simulink model "swcStopLightsMgr"  (R2022b)
settings: Solver=FixedStepDiscrete  StartTime=0  StopTime=10.0  FixedStep=0.01  RelTol=1e-3
values from neighbouring files (symbols this model uses):
  C1d_stopLightsMgrPriorityTable = Simulink.Parameter    [swcStopLightsMgr_defineIntCalibs.m]
  C_stopLightsEmergencyPeriod = Simulink.Parameter    [swcStopLightsMgr_defineIntCalibs.m]
  C_stopLightsSpeedThresholdSafety = Simulink.Parameter    [swcBrakePedalSignalingApp_defineIntCalibs.m]    (also in swcStopLightsMgr_defineIntCalibs.m)
  CONST_TWO = uint8(2)    [swcStopLightsMgr_defineIntParams.m]
  failureAlert = Simulink.Signal    [swcStopLightsMgr_defineIntCalibs.m]
  Init_FailureAlert = struct('valueState',ValueState.VALUE_STATE_VALID,'failureAlert',FailureAlert.FAILURE_ALERT_NO,'occurrence',uint8(0))    [swcStopLightsMgr_defineIntParams.m]
  Init_lightRequest = struct('Left_lightState',StopLightStateID.STOP_LIGHT_STATE_ID_OFF,'Right_lightState',StopLightStateID.STOP_LIGHT_STATE_ID_OFF,'Middle_lightState',StopLightStateID.STOP_LIGHT_STATE_ID_OFF)    [swcStopLightsMgr_defineIntParams.m]
  Init_setLight = struct('usageId',uint8(0),'LightOut',Init_lightRequest,'requestedPattern',StopLightsPatternID.STOP_LIGHTS_PATTERN_ID_OFF,'isStopLightsOn',false,'BrakeLampStatus',CANBrakeLampStatus.CANBRAKELAMPSTATUS_OFF)    [swcStopLightsMgr_defineIntParams.m]
  Init_StopLightsEvent = struct('valueState',ValueState.VALUE_STATE_VALID,'usageId',uint8(0),'requestedPattern',StopLightsPatternID.STOP_LIGHTS_PATTERN_ID_OFF)    [swcStopLightsMgr_defineIntParams.m]
  Init_switchStopLightState = struct('lightState',StopLightStateID.STOP_LIGHT_STATE_ID_OFF)    [swcStopLightsMgr_defineIntParams.m]
  OCCURRENCE_FALSE = uint8(0)    [swcStopLightsMgr_defineIntParams.m]
  OCCURRENCE_TRUE = uint8(1)    [swcStopLightsMgr_defineIntParams.m]
  PeriodResolution = uint8(20)    [swcStopLightsMgr_defineIntParams.m]
  POWER_AUTHORIZER = uint8(1)    [swcStopLightsMgr_defineIntParams.m]
  STEP_StopLightsMgr = 0.01    [swcStopLightsMgr_defineIntParams.m]
  STOPLIGHTS_IDX = uint8(64)    [swcStopLightsMgr_defineIntParams.m]
  STOPLIGHTS_USAGES_OUTSIDE_WARNING_ON_STRONG_BRAKING = uint8(18)    [swcStopLightsMgr_defineIntParams.m]
  TENMs = uint8(10)    [swcStopLightsMgr_defineIntParams.m]
  USAGEID_DEF = uint8(255)    [swcStopLightsMgr_defineIntParams.m]
  USAGEID_MIN = uint8(0)    [swcStopLightsMgr_defineIntParams.m]
undefined symbols (not defined in the file or in its folder): CANBrakeLampStatus, CANStopLampDiagnosis, occurrence, StopLampDiagnosis, UsageAction, valueState, ValueState
libraries: Ampere_Library x27, simulink x3, KPIT_eBody_Lib_Lighting x1
(part 1 of 2)
settings Model: ModifiedByFormat=Smrithi Pai  Creator=Smrithi Pai  LastModifiedBy=Smrithi Pai
settings DataIOCC: SaveOutput=off  SignalLogging=off  DSMLogging=off  SaveTime=off  ReturnWorkspaceOutputs=off
settings OptimizationCC: DefaultParameterBehavior=Inlined  EnhancedBackFolding=on  PassReuseOutputArgsAs=Individual arguments  ZeroExternalMemoryAtStartup=off  ZeroInternalMemoryAtStartup=off  LifeSpan=inf  OptimizeBlockOrder=speed  DifferentSizesBufferReuse=on  OptimizationCustomize=off  EfficientTunableParamExpr=on
settings DebuggingCC: SignalInfNanChecking=error  SignalRangeChecking=error  ReadBeforeWriteMsg=EnableAllAsError  WriteAfterWriteMsg=EnableAllAsError  WriteAfterReadMsg=EnableAllAsError  AlgebraicLoopMsg=error  ArtificialAlgebraicLoopMsg=error  SaveWithDisabledLinksMsg=error  SaveWithParameterizedLinksMsg=error  BlockPriorityViolationMsg=error  MinStepSizeMsg=error  TimeAdjustmentMsg=warning  SolverPrmCheckMsg=error  MultiTaskRateTransMsg=warning  SingleTaskRateTransMsg=warning  TasksWithSamePriorityMsg=error  SigSpecEnsureSampleTimeMsg=error  CheckMatrixSingularityMsg=error  IntegerOverflowMsg=error  ParameterUnderflowMsg=error  ParameterPrecisionLossMsg=error  ParameterTunabilityLossMsg=error  FixptConstUnderflowMsg=warning  FixptConstOverflowMsg=warning  FixptConstPrecisionLossMsg=warning  UnderSpecifiedDataTypeMsg=error  UnnecessaryDatatypeConvMsg=warning  VectorMatrixConversionMsg=error  UnconnectedInputMsg=error  UnconnectedOutputMsg=error  UnconnectedLineMsg=error  FrameProcessingCompatibilityMsg=warning  UniqueDataStoreMsg=error  BusObjectLabelMismatch=error  RootOutportRequireBusObject=error  AssertControl=DisableAll  ModelReferenceIOMsg=error  UnknownTsInhSupMsg=error  ModelReferenceDataLoggingMessage=error  StateNameClashWarn=warning  StrictBusMsg=ErrorOnBusTreatedAsVector  NonBusSignalsTreatedAsBus=error  SFUnusedDataAndEventsDiag=error  SFInvalidInputDataAccessInChartInitDiag=error  SFTransitionOutsideNaturalParentDiag=error  SFUnreachableExecutionPathDiag=error  SFUndirectedBroadcastEventsDiag=error  SFTransitionActionBeforeConditionDiag=error  SFTemporalDelaySmallerThanSampleTimeDiag=error  SFSelfTransitionDiag=error  UnderSpecifiedDimensionMsg=error  VariantConditionMismatch=error
settings ModelReferenceCC: EnableRefExpFcnMdlSchedulingChecks=on  ModelReferenceNumInstancesAllowed=Single
settings SFSimCC: SimIntegrity=alwaysOn  SimGenImportedTypeDefs=on  CompileTimeRecursionLimit=0  EnableRuntimeRecursion=off  MATLABDynamicMemAlloc=off
settings RTWCC: Description=AUTOSAR  SystemTargetFile=autosar.tlc  GenCodeOnly=on  TemplateMakefile=ert_default_tmf
settings CodeAppCC: ForceParamTrailComments=on  IgnoreCustomStorageClasses=off  OperatorAnnotations=on  SimulinkDataObjDesc=on  SFDataObjDesc=on  InsertBlockDesc=on
settings STFCustomTargetCC: TargetLangStandard=C99 (ISO)  MultiwordLength=256  ParMdlRefBuildCompliant=on  CompOptLevelCompliant=on  IncludeMdlTerminateFcn=off  CombineOutputUpdateFcns=on  SuppressErrorStatus=on  ERTCustomFileBanners=on  SupportNonFinite=off  SupportComplex=off  SupportContinuousTime=off  SupportNonInlinedSFcns=off  RemoveResetFunc=on  MATLABClassNameForMDSCustomization=Simulink.SoftwareTarget.ERTCustomization  AutosarCompliant=on  UseToolchainInfoCompliant=on  LookupTableObjectStructAxisOrder=2,1,3,4,...  LUTObjectStructOrderEvenSpacing=Size,Table,Breakpoints  SystemTargetFile=autosar.tlc
settings ERTTargetCC: TargetLangStandard=C99 (ISO)  ConcurrentExecutionCompliant=off  IncludeMdlTerminateFcn=off  SuppressErrorStatus=on  SupportNonFinite=off  SupportComplex=off  ModelStepFunctionPrototypeControlCompliant=off  CPPClassGenCompliant=off  AutosarCompliant=on  LookupTableObjectStructAxisOrder=2,1,3,4,...  LUTObjectStructOrderEvenSpacing=Size,Table,Breakpoints  InlinedParameterPlacement=NonHierarchical  ERTCustomFileTemplate=example_file_process.tlc

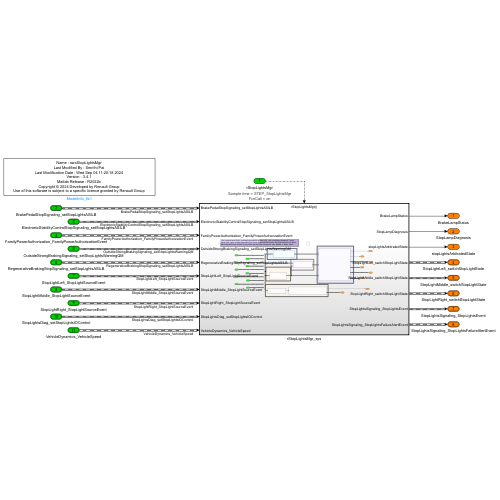
[thumbnail: Simulink's stored preview of the top-level diagram]
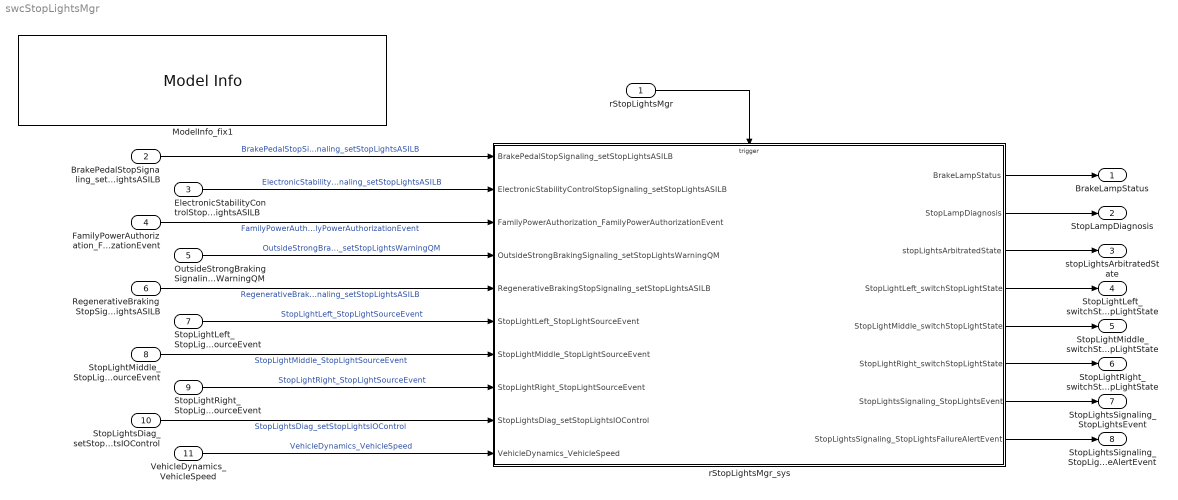
== system swcStopLightsMgr ==
  rStopLightsMgr : Inport  SampleTime=STEP_StopLightsMgr  OutputFunctionCall=on
      settings: AttributesFormatString=Sample time = %<SampleTime>\nFcnCall = %<OutputFunctionCall>
  BrakePedalStopSignaling_setStopLightsASILB : Inport  Port=2  OutDataTypeStr=Bus: setStopLightsASILB  PortDimensions=1  BusOutputAsStruct=on
  ElectronicStabilityControlStopSignaling_setStopLightsASILB : Inport  Port=3  OutDataTypeStr=Bus: setStopLightsASILB  PortDimensions=1  BusOutputAsStruct=on
  FamilyPowerAuthorization_FamilyPowerAuthorizationEvent : Inport  Port=4  OutDataTypeStr=Bus: FamilyPowerAuthorizationEvent  PortDimensions=1  BusOutputAsStruct=on
  OutsideStrongBrakingSignaling_setStopLightsWarningQM : Inport  Port=5  OutDataTypeStr=Bus: setStopLightsWarningQM  PortDimensions=1  BusOutputAsStruct=on
  RegenerativeBrakingStopSignaling_setStopLightsASILB : Inport  Port=6  OutDataTypeStr=Bus: setStopLightsASILB  PortDimensions=1  BusOutputAsStruct=on
  StopLightLeft_StopLightSourceEvent : Inport  Port=7  OutDataTypeStr=Bus: StopLightSourceEvent  PortDimensions=1  BusOutputAsStruct=on
  StopLightMiddle_StopLightSourceEvent : Inport  Port=8  OutDataTypeStr=Bus: StopLightSourceEvent  PortDimensions=1  BusOutputAsStruct=on
  StopLightRight_StopLightSourceEvent : Inport  Port=9  OutDataTypeStr=Bus: StopLightSourceEvent  PortDimensions=1  BusOutputAsStruct=on
  StopLightsDiag_setStopLightsIOControl : Inport  Port=10  OutDataTypeStr=Bus: setStopLightsIOControl  PortDimensions=1  BusOutputAsStruct=on
  VehicleDynamics_VehicleSpeed : Inport  Port=11  OutDataTypeStr=Bus: VehicleSpeed  PortDimensions=1  BusOutputAsStruct=on
  ModelInfo_fix1 : simulink/Model-Wide Utilities/Model Info  Frame=on  DisplayStringWithTags=|  HorizontalTextAlignment=Center  LeftAlignmentValue=0.5
      | Name : %<ModelName>
      | Last Modified By : %<LastModifiedBy>
      | Last Modification Date : %<LastModificationDate>
      | Version : %<ModelVersion>
      | Matlab Release : R2022b
      | Copyright © 2024 Developed by Renault Group
      | Use of this software is subject to a specific licence granted by Renault Group
  rStopLightsMgr_sys : Subsystem
  BrakeLampStatus : Outport  OutDataTypeStr=Enum: CANBrakeLampStatus  PortDimensions=1
  StopLampDiagnosis : Outport  Port=2  OutDataTypeStr=Enum: CANStopLampDiagnosis  PortDimensions=1
  stopLightsArbitratedState : Outport  Port=3  OutDataTypeStr=boolean  PortDimensions=1
  StopLightLeft_switchStopLightState : Outport  Port=4  OutDataTypeStr=Bus: switchStopLightState  PortDimensions=1  BusOutputAsStruct=on
  StopLightMiddle_switchStopLightState : Outport  Port=5  OutDataTypeStr=Bus: switchStopLightState  PortDimensions=1  BusOutputAsStruct=on
  StopLightRight_switchStopLightState : Outport  Port=6  OutDataTypeStr=Bus: switchStopLightState  PortDimensions=1  BusOutputAsStruct=on
  StopLightsSignaling_StopLightsEvent : Outport  Port=7  OutDataTypeStr=Bus: StopLightsEvent  PortDimensions=1  BusOutputAsStruct=on
  StopLightsSignaling_StopLightsFailureAlertEvent : Outport  Port=8  OutDataTypeStr=Bus: StopLightsFailureAlertEvent  PortDimensions=1  BusOutputAsStruct=on
  wires:
  rStopLightsMgr_sys/8(StopLightsSignaling_StopLightsFailureAlertEvent) -> StopLightsSignaling_StopLightsFailureAlertEvent/1
  rStopLightsMgr_sys/5(StopLightMiddle_switchStopLightState) -> StopLightMiddle_switchStopLightState/1
  rStopLightsMgr_sys/4(StopLightLeft_switchStopLightState) -> StopLightLeft_switchStopLightState/1
  rStopLightsMgr_sys/2(StopLampDiagnosis) -> StopLampDiagnosis/1
  rStopLightsMgr_sys/7(StopLightsSignaling_StopLightsEvent) -> StopLightsSignaling_StopLightsEvent/1
  rStopLightsMgr/1 -> rStopLightsMgr_sys/Trigger
  ElectronicStabilityControlStopSignaling_setStopLightsASILB/1 -> rStopLightsMgr_sys/2(ElectronicStabilityControlStopSignaling_setStopLightsASILB)  "ElectronicStabilityControlStopSignaling_setStopLightsASILB"
  FamilyPowerAuthorization_FamilyPowerAuthorizationEvent/1 -> rStopLightsMgr_sys/3(FamilyPowerAuthorization_FamilyPowerAuthorizationEvent)  "FamilyPowerAuthorization_FamilyPowerAuthorizationEvent"
  rStopLightsMgr_sys/3(stopLightsArbitratedState) -> stopLightsArbitratedState/1
  RegenerativeBrakingStopSignaling_setStopLightsASILB/1 -> rStopLightsMgr_sys/5(RegenerativeBrakingStopSignaling_setStopLightsASILB)  "RegenerativeBrakingStopSignaling_setStopLightsASILB"
  rStopLightsMgr_sys/1(BrakeLampStatus) -> BrakeLampStatus/1
  BrakePedalStopSignaling_setStopLightsASILB/1 -> rStopLightsMgr_sys/1(BrakePedalStopSignaling_setStopLightsASILB)  "BrakePedalStopSignaling_setStopLightsASILB"
  OutsideStrongBrakingSignaling_setStopLightsWarningQM/1 -> rStopLightsMgr_sys/4(OutsideStrongBrakingSignaling_setStopLightsWarningQM)  "OutsideStrongBrakingSignaling_setStopLightsWarningQM"
  StopLightLeft_StopLightSourceEvent/1 -> rStopLightsMgr_sys/6(StopLightLeft_StopLightSourceEvent)  "StopLightLeft_StopLightSourceEvent"
  StopLightMiddle_StopLightSourceEvent/1 -> rStopLightsMgr_sys/7(StopLightMiddle_StopLightSourceEvent)  "StopLightMiddle_StopLightSourceEvent"
  StopLightRight_StopLightSourceEvent/1 -> rStopLightsMgr_sys/8(StopLightRight_StopLightSourceEvent)  "StopLightRight_StopLightSourceEvent"
  StopLightsDiag_setStopLightsIOControl/1 -> rStopLightsMgr_sys/9(StopLightsDiag_setStopLightsIOControl)  "StopLightsDiag_setStopLightsIOControl"
  rStopLightsMgr_sys/6(StopLightRight_switchStopLightState) -> StopLightRight_switchStopLightState/1
  VehicleDynamics_VehicleSpeed/1 -> rStopLightsMgr_sys/10(VehicleDynamics_VehicleSpeed)  "VehicleDynamics_VehicleSpeed"

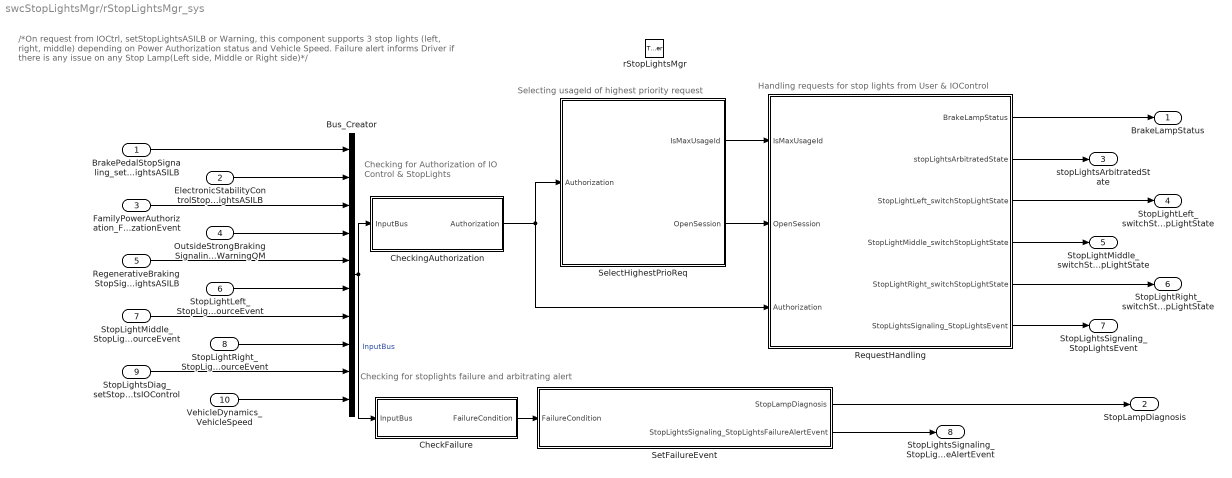
== system swcStopLightsMgr/rStopLightsMgr_sys ==
  note: Checking for Authorization of
      | IO Control & StopLights
  note: Handling requests for stop lights from User & IOControl
  note: Checking for stoplights failure and arbitrating alert
  note: Selecting usageId of highest priority request
  note: /*On request from IOCtrl, setStopLightsASILB or Warning, this component supports 3 stop lights (left, right, middle) depending on Power Authorization status and Vehicle Speed. Failure alert informs Driver if there is any issue on any Stop Lamp(Left side, Middle or Right side)*/
  BrakePedalStopSignaling_setStopLightsASILB : Inport
  ElectronicStabilityControlStopSignaling_setStopLightsASILB : Inport  Port=2
  FamilyPowerAuthorization_FamilyPowerAuthorizationEvent : Inport  Port=3
  OutsideStrongBrakingSignaling_setStopLightsWarningQM : Inport  Port=4
  RegenerativeBrakingStopSignaling_setStopLightsASILB : Inport  Port=5
  StopLightLeft_StopLightSourceEvent : Inport  Port=6
  StopLightMiddle_StopLightSourceEvent : Inport  Port=7
  StopLightRight_StopLightSourceEvent : Inport  Port=8
  StopLightsDiag_setStopLightsIOControl : Inport  Port=9
  VehicleDynamics_VehicleSpeed : Inport  Port=10
  rStopLightsMgr : TriggerPort  TriggerType=function-call  VariantControl=(inherit)  SampleTimeType=periodic  SampleTime=-1  PortDimensions=1
      settings: AttributesFormatString=%<StatesWhenEnabling>\n
  Bus_Creator : BusCreator  Inputs=10
  CheckFailure : Subsystem  Description=|  TreatAsAtomicUnit=on
      | StopLightsMgr_Req_41
      | StopLightsMgr_Req_43
      | StopLightsMgr_Req_100333
  CheckingAuthorization : Subsystem  Description=StopLightsMgr_Req_22  TreatAsAtomicUnit=on
  RequestHandling : Subsystem  Description=<binary blob, 146 chars, not shown>  TreatAsAtomicUnit=on
  SelectHighestPrioReq : Subsystem  Description=StopLightsMgr_Req_22  TreatAsAtomicUnit=on
  SetFailureEvent : Subsystem  Description=|  TreatAsAtomicUnit=on
      | StopLightsMgr_Req_40
      | StopLightsMgr_Req_44
      | StopLightsMgr_Req_48
      | StopLightsMgr_Req_49
  BrakeLampStatus : Outport  InitialOutput=CANBrakeLampStatus.CANBRAKELAMPSTATUS_OFF
      settings: AttributesFormatString=Init = %<InitialOutput>\n
  StopLampDiagnosis : Outport  Port=2  InitialOutput=CANStopLampDiagnosis.CANSTOPLAMPDIAGNOSIS_NO_FAILURE
      settings: AttributesFormatString=Init = %<InitialOutput>\n
  stopLightsArbitratedState : Outport  Port=3  InitialOutput=false
      settings: AttributesFormatString=Init = %<InitialOutput>\n
  StopLightLeft_switchStopLightState : Outport  Port=4  InitialOutput=Init_switchStopLightState
      settings: AttributesFormatString=Init = %<InitialOutput>\n
  StopLightMiddle_switchStopLightState : Outport  Port=5  InitialOutput=Init_switchStopLightState
      settings: AttributesFormatString=Init = %<InitialOutput>\n
  StopLightRight_switchStopLightState : Outport  Port=6  InitialOutput=Init_switchStopLightState
      settings: AttributesFormatString=Init = %<InitialOutput>\n
  StopLightsSignaling_StopLightsEvent : Outport  Port=7  InitialOutput=Init_StopLightsEvent
      settings: AttributesFormatString=Init = %<InitialOutput>\n
  StopLightsSignaling_StopLightsFailureAlertEvent : Outport  Port=8  InitialOutput=Init_FailureAlert
      settings: AttributesFormatString=Init = %<InitialOutput>\n
  wires:
  BrakePedalStopSignaling_setStopLightsASILB/1 -> Bus_Creator/1
  ElectronicStabilityControlStopSignaling_setStopLightsASILB/1 -> Bus_Creator/2
  FamilyPowerAuthorization_FamilyPowerAuthorizationEvent/1 -> Bus_Creator/3
  OutsideStrongBrakingSignaling_setStopLightsWarningQM/1 -> Bus_Creator/4
  RegenerativeBrakingStopSignaling_setStopLightsASILB/1 -> Bus_Creator/5
  StopLightLeft_StopLightSourceEvent/1 -> Bus_Creator/6
  StopLightMiddle_StopLightSourceEvent/1 -> Bus_Creator/7
  StopLightRight_StopLightSourceEvent/1 -> Bus_Creator/8
  StopLightsDiag_setStopLightsIOControl/1 -> Bus_Creator/9
  VehicleDynamics_VehicleSpeed/1 -> Bus_Creator/10
  RequestHandling/1(BrakeLampStatus) -> BrakeLampStatus/1
  SelectHighestPrioReq/1(IsMaxUsageId) -> RequestHandling/1(IsMaxUsageId)
  CheckingAuthorization/1(Authorization) -> RequestHandling/3(Authorization), SelectHighestPrioReq/1(Authorization)
  RequestHandling/2(stopLightsArbitratedState) -> stopLightsArbitratedState/1
  RequestHandling/3(StopLightLeft_switchStopLightState) -> StopLightLeft_switchStopLightState/1
  RequestHandling/4(StopLightMiddle_switchStopLightState) -> StopLightMiddle_switchStopLightState/1
  RequestHandling/5(StopLightRight_switchStopLightState) -> StopLightRight_switchStopLightState/1
  RequestHandling/6(StopLightsSignaling_StopLightsEvent) -> StopLightsSignaling_StopLightsEvent/1
  SetFailureEvent/1(StopLampDiagnosis) -> StopLampDiagnosis/1
  SetFailureEvent/2(StopLightsSignaling_StopLightsFailureAlertEvent) -> StopLightsSignaling_StopLightsFailureAlertEvent/1
  Bus_Creator/1 -> CheckFailure/1(InputBus), CheckingAuthorization/1(InputBus)  "InputBus"
  CheckFailure/1(FailureCondition) -> SetFailureEvent/1(FailureCondition)
  SelectHighestPrioReq/2(OpenSession) -> RequestHandling/2(OpenSession)

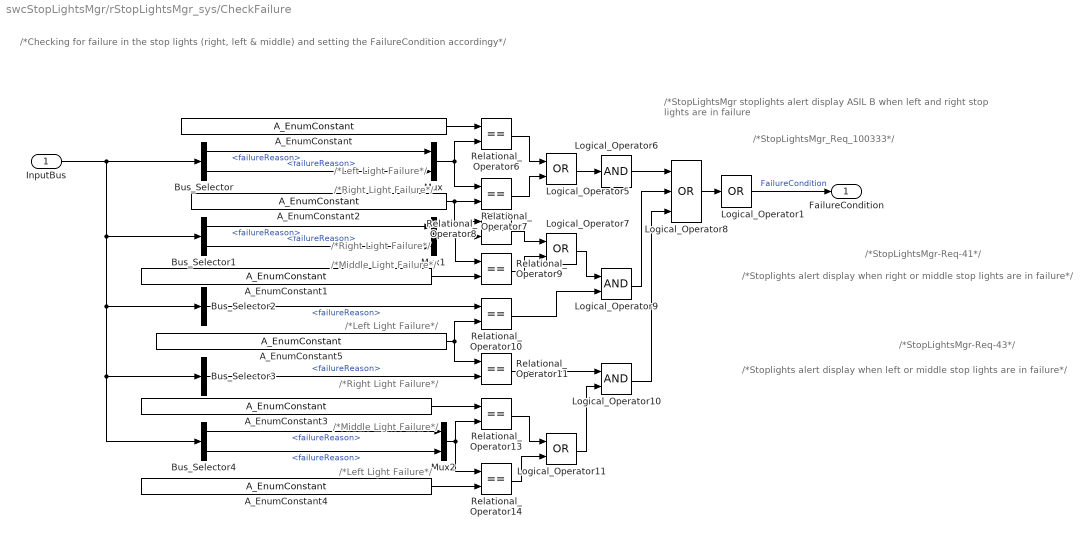
== system swcStopLightsMgr/rStopLightsMgr_sys/CheckFailure ==
  note: /*Left Light Failure*/
  note: /*Stoplights alert display when right or middle stop
      | lights are in failure*/
  note: /*StopLightsMgr stoplights alert display
      | ASIL B when left and right stop lights are in failure
  note: /*Stoplights alert display when left or middle stop lights
      | are in failure*/
  note: /*Right Light Failure*/
  note: /*Right Light Failure*/
  note: /*Middle Light Failure*/
  note: /*Left Light Failure*/
  note: /*Middle Light Failure*/
  note: /*Left Light Failure*/
  note: /*Right Light Failure*/
  note: /*StopLightsMgr_Req_100333*/
  note: /*StopLightsMgr-Req-41*/
  note: /*StopLightsMgr-Req-43*/
  note: /*Checking for failure in the stop lights (right, left & middle) and setting the FailureCondition accordingy*/
  InputBus : Inport
  A_EnumConstant : Ampere_Library/User_Defined_Libraries/Sources/A_EnumConstant  Tag=[LIB]  OutDataTypeStr=Enum: LightSourceFailureReason  EnumVal=LIGHT_SOURCE_FAILURE_REASON_SC_TO_GND
      settings: AttributesFormatString=Enum: LightSourceFailureReason
  A_EnumConstant1 : Ampere_Library/User_Defined_Libraries/Sources/A_EnumConstant  Tag=[LIB]  OutDataTypeStr=Enum: LightSourceFailureReason  EnumVal=LIGHT_SOURCE_FAILURE_REASON_SC_TO_GND
      settings: AttributesFormatString=Enum: LightSourceFailureReason
  A_EnumConstant2 : Ampere_Library/User_Defined_Libraries/Sources/A_EnumConstant  Tag=[LIB]  OutDataTypeStr=Enum: LightSourceFailureReason  EnumVal=LIGHT_SOURCE_FAILURE_REASON_OPEN_CIRCUIT
      settings: AttributesFormatString=Enum: LightSourceFailureReason
  A_EnumConstant3 : Ampere_Library/User_Defined_Libraries/Sources/A_EnumConstant  Tag=[LIB]  OutDataTypeStr=Enum: LightSourceFailureReason  EnumVal=LIGHT_SOURCE_FAILURE_REASON_OPEN_CIRCUIT
      settings: AttributesFormatString=Enum: LightSourceFailureReason
  A_EnumConstant4 : Ampere_Library/User_Defined_Libraries/Sources/A_EnumConstant  Tag=[LIB]  OutDataTypeStr=Enum: LightSourceFailureReason  EnumVal=LIGHT_SOURCE_FAILURE_REASON_SC_TO_GND
      settings: AttributesFormatString=Enum: LightSourceFailureReason
  A_EnumConstant5 : Ampere_Library/User_Defined_Libraries/Sources/A_EnumConstant  Tag=[LIB]  OutDataTypeStr=Enum: LightSourceFailureReason  EnumVal=LIGHT_SOURCE_FAILURE_REASON_NONE
      settings: AttributesFormatString=Enum: LightSourceFailureReason
  Bus_Selector : BusSelector  OutputSignals=StopLightLeft_StopLightSourceEvent.failureReason,StopLightRight_StopLightSourceEvent.failureReason
  Bus_Selector1 : BusSelector  OutputSignals=StopLightMiddle_StopLightSourceEvent.failureReason,StopLightRight_StopLightSourceEvent.failureReason
  Bus_Selector2 : BusSelector  OutputSignals=StopLightLeft_StopLightSourceEvent.failureReason
  Bus_Selector3 : BusSelector  OutputSignals=StopLightRight_StopLightSourceEvent.failureReason
  Bus_Selector4 : BusSelector  OutputSignals=StopLightMiddle_StopLightSourceEvent.failureReason,StopLightLeft_StopLightSourceEvent.failureReason
  Logical_Operator1 : Logic  Operator=OR  Inputs=1  OutDataTypeStr=boolean
  Logical_Operator10 : Logic  OutDataTypeStr=boolean
  Logical_Operator11 : Logic  Operator=OR  OutDataTypeStr=boolean
  Logical_Operator5 : Logic  Operator=OR  OutDataTypeStr=boolean
  Logical_Operator6 : Logic  Inputs=1  OutDataTypeStr=boolean
  Logical_Operator7 : Logic  Operator=OR  OutDataTypeStr=boolean
  Logical_Operator8 : Logic  Operator=OR  Inputs=3  OutDataTypeStr=boolean
  Logical_Operator9 : Logic  OutDataTypeStr=boolean
  Mux : Mux  Inputs=2
  Mux1 : Mux  Inputs=2
  Mux2 : Mux  Inputs=2
  Relational_Operator{6..11,13..14} (8 alike) : RelationalOperator  Operator===  OutDataTypeStr=boolean  RndMeth=Zero
  FailureCondition : Outport
  wires:
  Relational_Operator11/1 -> Logical_Operator10/1
  Mux/1 -> Relational_Operator6/2, Relational_Operator7/1
  Bus_Selector4/1 -> Mux2/1  "<failureReason>"
  Bus_Selector1/2 -> Mux1/2  "<failureReason>"
  Logical_Operator6/1 -> Logical_Operator8/1
  InputBus/1 -> Bus_Selector/1, Bus_Selector4/1, Bus_Selector3/1, Bus_Selector2/1, Bus_Selector1/1
  Logical_Operator9/1 -> Logical_Operator8/2
  Relational_Operator7/1 -> Logical_Operator5/2
  Mux2/1 -> Relational_Operator14/1, Relational_Operator13/2
  Bus_Selector/2 -> Mux/2  "<failureReason>"
  A_EnumConstant2/1 -> Relational_Operator8/1, Relational_Operator7/2
  A_EnumConstant/1 -> Relational_Operator6/1
  Bus_Selector3/1 -> Relational_Operator11/2  "<failureReason>"
  Relational_Operator8/1 -> Logical_Operator7/1
  Mux1/1 -> Relational_Operator9/1, Relational_Operator8/2
  Logical_Operator5/1 -> Logical_Operator6/1
  A_EnumConstant1/1 -> Relational_Operator9/2
  A_EnumConstant5/1 -> Relational_Operator11/1, Relational_Operator10/2
  Bus_Selector2/1 -> Relational_Operator10/1  "<failureReason>"
  A_EnumConstant3/1 -> Relational_Operator13/1
  Bus_Selector/1 -> Mux/1  "<failureReason>"
  Relational_Operator10/1 -> Logical_Operator9/2
  Relational_Operator6/1 -> Logical_Operator5/1
  Bus_Selector1/1 -> Mux1/1  "<failureReason>"
  Relational_Operator9/1 -> Logical_Operator7/2
  Logical_Operator11/1 -> Logical_Operator10/2
  A_EnumConstant4/1 -> Relational_Operator14/2
  Bus_Selector4/2 -> Mux2/2  "<failureReason>"
  Logical_Operator10/1 -> Logical_Operator8/3
  Logical_Operator7/1 -> Logical_Operator9/1
  Relational_Operator14/1 -> Logical_Operator11/2
  Relational_Operator13/1 -> Logical_Operator11/1
  Logical_Operator8/1 -> Logical_Operator1/1
  Logical_Operator1/1 -> FailureCondition/1  "FailureCondition"

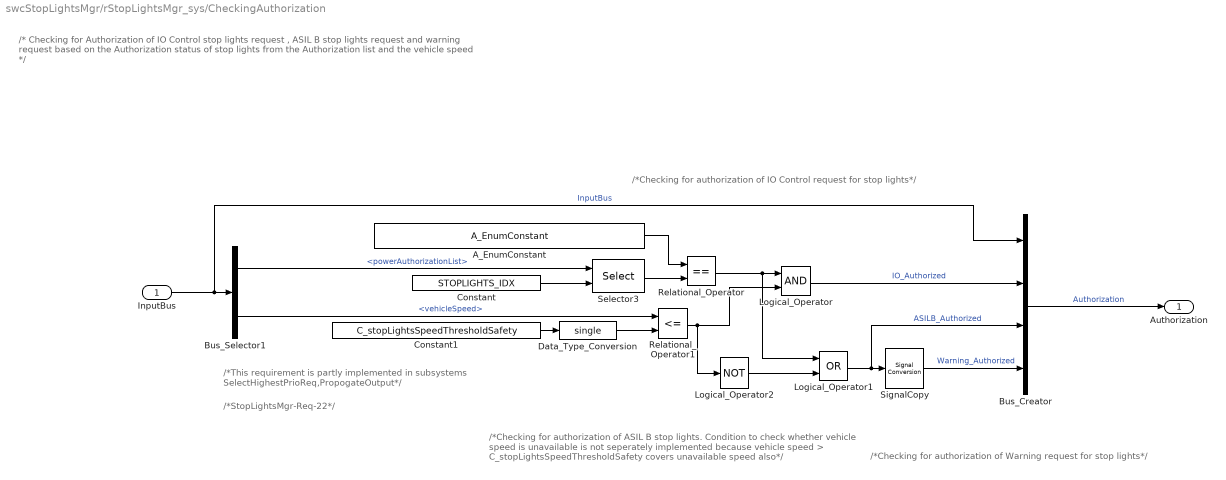
== system swcStopLightsMgr/rStopLightsMgr_sys/CheckingAuthorization ==
  note: /*Checking for authorization of ASIL B stop lights. Condition to check whether vehicle speed is unavailable is not seperately implemented because vehicle speed > C_stopLightsSpeedThresholdSafety covers unavailable speed also*/
  note: /*StopLightsMgr-Req-22*/
  note: /*This requirement is partly implemented in subsystems SelectHighestPrioReq,PropogateOutput*/
  note: /*Checking for authorization of IO Control request for stop lights*/
  note: /*Checking for authorization of Warning request for stop lights*/
  note: /* Checking for Authorization of IO Control stop lights request , ASIL B stop lights request and warning request based on the Authorization status of stop lights from the Authorization list and the vehicle speed */
  InputBus : Inport
  A_EnumConstant : Ampere_Library/User_Defined_Libraries/Sources/A_EnumConstant  Tag=[LIB]  OutDataTypeStr=Enum: PowerAuthorizationStatus  EnumVal=POWERAUTHORIZATIONSTATUS_AUTHORIZED
      settings: AttributesFormatString=Enum: PowerAuthorizationStatus
  Bus_Creator : BusCreator  Inputs=4
  Bus_Selector1 : BusSelector  OutputSignals=FamilyPowerAuthorization_FamilyPowerAuthorizationEvent.powerAuthorizationList,VehicleDynamics_VehicleSpeed.vehicleSpeed
  Constant : Constant  Value=STOPLIGHTS_IDX
  Constant1 : Constant  Value=C_stopLightsSpeedThresholdSafety
  Data_Type_Conversion : DataTypeConversion  OutDataTypeStr=single  SaturateOnIntegerOverflow=off
  Logical_Operator : Logic  OutDataTypeStr=boolean
  Logical_Operator1 : Logic  Operator=OR  OutDataTypeStr=boolean
  Logical_Operator2 : Logic  Operator=NOT  OutDataTypeStr=boolean
  Relational_Operator : RelationalOperator  Operator===  OutDataTypeStr=boolean  RndMeth=Zero
  Relational_Operator1 : RelationalOperator  Operator=<=  OutDataTypeStr=boolean  RndMeth=Zero
  Selector3 : Selector  IndexMode=Zero-based  InputPortWidth=450  IndexOptions=Index vector (port)  Indices=[1 3]  OutputSizes=1
      settings: AttributesFormatString=%<IndexMode>\n
  SignalCopy : SignalConversion  OverrideOpt=off
  Authorization : Outport
  wires:
  Bus_Selector1/1 -> Selector3/1  "<powerAuthorizationList>"
  A_EnumConstant/1 -> Relational_Operator/1
  Constant/1 -> Selector3/2
  Selector3/1 -> Relational_Operator/2
  InputBus/1 -> Bus_Creator/1, Bus_Selector1/1  "InputBus"
  Constant1/1 -> Data_Type_Conversion/1
  Data_Type_Conversion/1 -> Relational_Operator1/2
  Relational_Operator1/1 -> Logical_Operator2/1, Logical_Operator/2
  Bus_Selector1/2 -> Relational_Operator1/1  "<vehicleSpeed>"
  Relational_Operator/1 -> Logical_Operator/1, Logical_Operator1/1
  Logical_Operator2/1 -> Logical_Operator1/2
  Logical_Operator/1 -> Bus_Creator/2  "IO_Authorized"
  Logical_Operator1/1 -> Bus_Creator/3, SignalCopy/1  "ASILB_Authorized"
  SignalCopy/1 -> Bus_Creator/4  "Warning_Authorized"
  Bus_Creator/1 -> Authorization/1  "Authorization"

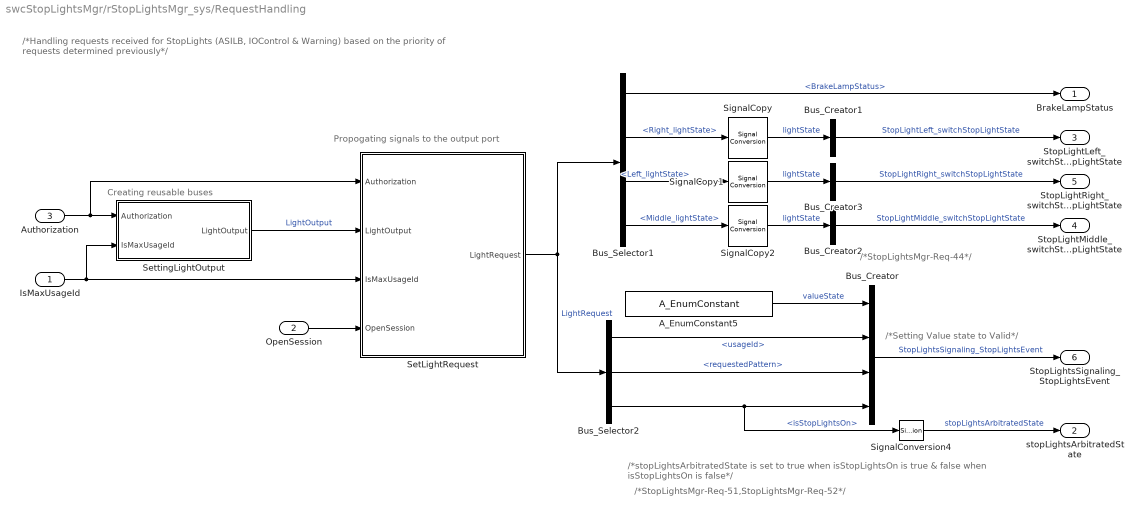
== system swcStopLightsMgr/rStopLightsMgr_sys/RequestHandling ==
  note: Propogating signals to the output port
  note: /*Setting Value state to Valid*/
  note: /*stopLightsArbitratedState is set to true when isStopLightsOn is true & false when isStopLightsOn is false*/
  note: /*StopLightsMgr-Req-44*/
  note: /*Handling requests received for StopLights (ASILB, IOControl & Warning) based on the priority of requests determined previously*/
  note: /*StopLightsMgr-Req-51,StopLightsMgr-Req-52*/
  note: Creating reusable buses
  IsMaxUsageId : Inport
  OpenSession : Inport  Port=2
  Authorization : Inport  Port=3
  A_EnumConstant5 : Ampere_Library/User_Defined_Libraries/Sources/A_EnumConstant  Tag=[LIB]  OutDataTypeStr=Enum: ValueState  EnumVal=VALUE_STATE_VALID
      settings: AttributesFormatString=Enum: ValueState
  Bus_Creator : BusCreator  Inputs='valueState','usageId','requestedPattern','isStopLightsOn'  OutDataTypeStr=Bus: StopLightsEvent  NonVirtualBus=on
  Bus_Creator1 : BusCreator  Inputs=lightState  OutDataTypeStr=Bus: switchStopLightState  NonVirtualBus=on
  Bus_Creator2 : BusCreator  Inputs=lightState  OutDataTypeStr=Bus: switchStopLightState  NonVirtualBus=on
  Bus_Creator3 : BusCreator  Inputs=lightState  OutDataTypeStr=Bus: switchStopLightState  NonVirtualBus=on
  Bus_Selector1 : BusSelector  OutputSignals=BrakeLampStatus,LightOut.Right_lightState,LightOut.Left_lightState,LightOut.Middle_lightState
  Bus_Selector2 : BusSelector  OutputSignals=usageId,requestedPattern,isStopLightsOn
  SetLightRequest : Subsystem  TreatAsAtomicUnit=on
  SettingLightOutput : Subsystem  Description=<binary blob, 196 chars, not shown>  TreatAsAtomicUnit=on
  SignalConversion4 : SignalConversion  OverrideOpt=off
  SignalCopy : SignalConversion  OverrideOpt=off
  SignalCopy1 : SignalConversion  OverrideOpt=off
  SignalCopy2 : SignalConversion  OverrideOpt=off
  BrakeLampStatus : Outport
  stopLightsArbitratedState : Outport  Port=2
  StopLightLeft_switchStopLightState : Outport  Port=3
  StopLightMiddle_switchStopLightState : Outport  Port=4
  StopLightRight_switchStopLightState : Outport  Port=5
  StopLightsSignaling_StopLightsEvent : Outport  Port=6
  wires:
  SetLightRequest/1(LightRequest) -> Bus_Selector1/1, Bus_Selector2/1  "LightRequest"
  Bus_Creator1/1 -> StopLightLeft_switchStopLightState/1  "StopLightLeft_switchStopLightState"
  Bus_Creator2/1 -> StopLightMiddle_switchStopLightState/1  "StopLightMiddle_switchStopLightState"
  Bus_Creator3/1 -> StopLightRight_switchStopLightState/1  "StopLightRight_switchStopLightState"
  SignalCopy1/1 -> Bus_Creator3/1  "lightState"
  Bus_Selector2/1 -> Bus_Creator/2  "<usageId>"
  Bus_Selector2/3 -> SignalConversion4/1, Bus_Creator/4  "<isStopLightsOn>"
  A_EnumConstant5/1 -> Bus_Creator/1  "valueState"
  Bus_Creator/1 -> StopLightsSignaling_StopLightsEvent/1  "StopLightsSignaling_StopLightsEvent"
  Bus_Selector2/2 -> Bus_Creator/3  "<requestedPattern>"
  SignalCopy2/1 -> Bus_Creator2/1  "lightState"
  SignalCopy/1 -> Bus_Creator1/1  "lightState"
  SettingLightOutput/1(LightOutput) -> SetLightRequest/2(LightOutput)  "LightOutput"
  SignalConversion4/1 -> stopLightsArbitratedState/1  "stopLightsArbitratedState"
  Bus_Selector1/2 -> SignalCopy/1  "<Right_lightState>"
  Bus_Selector1/3 -> SignalCopy1/1  "<Left_lightState>"
  Bus_Selector1/4 -> SignalCopy2/1  "<Middle_lightState>"
  Bus_Selector1/1 -> BrakeLampStatus/1  "<BrakeLampStatus>"
  IsMaxUsageId/1 -> SettingLightOutput/2(IsMaxUsageId), SetLightRequest/3(IsMaxUsageId)
  OpenSession/1 -> SetLightRequest/4(OpenSession)
  Authorization/1 -> SetLightRequest/1(Authorization), SettingLightOutput/1(Authorization)

== system swcStopLightsMgr/rStopLightsMgr_sys/SelectHighestPrioReq ==
  note: Selecting the UsageID of the client which has the highest
      | priority
  note: /*This requirement is partly implemented in subsystems
      | CheckingAuthorization, PropogateOutput*/
  note: Selecting the Usage ID depending on the request received StopLights, IO Control or
      | Warning
  note: /*StopLightsMgr-Req-22*/
  note: /* In this subsystem ASILB, IOCtrl and warning priority selection(Selected_Priority) is done. If there is no request fromASILB, IOCTRL and warning then stop lamps will turn off*/
  Authorization : Inport
  Bus_Selector2 : BusSelector  OutputSignals=IO_Authorized,ASILB_Authorized,Warning_Authorized
  SelectRequestFromPriority : Subsystem
  SelectingRequest : Subsystem  TreatAsAtomicUnit=on
  IsMaxUsageId : Outport
  OpenSession : Outport  Port=2
  wires:
  SelectingRequest/1(Selected_usageId) -> SelectRequestFromPriority/1(Selected_usageId)  "Selected_usageId"
  SelectRequestFromPriority/1(IsMaxUsageId) -> IsMaxUsageId/1  "IsMaxUsageId"
  SelectingRequest/2(InputUsageID) -> SelectRequestFromPriority/2(InputUsageID)
  Authorization/1 -> Bus_Selector2/1, SelectingRequest/1(Authorization)
  Bus_Selector2/2 -> SelectingRequest/3(ASILB_Authorized)  "<ASILB_Authorized>"
  Bus_Selector2/3 -> SelectingRequest/4(Warning_Authorized)  "<Warning_Authorized>"
  SelectingRequest/3(OpenSession) -> OpenSession/1  "OpenSession"
  Bus_Selector2/1 -> SelectingRequest/2(IO_Authorized)  "<IO_Authorized>"

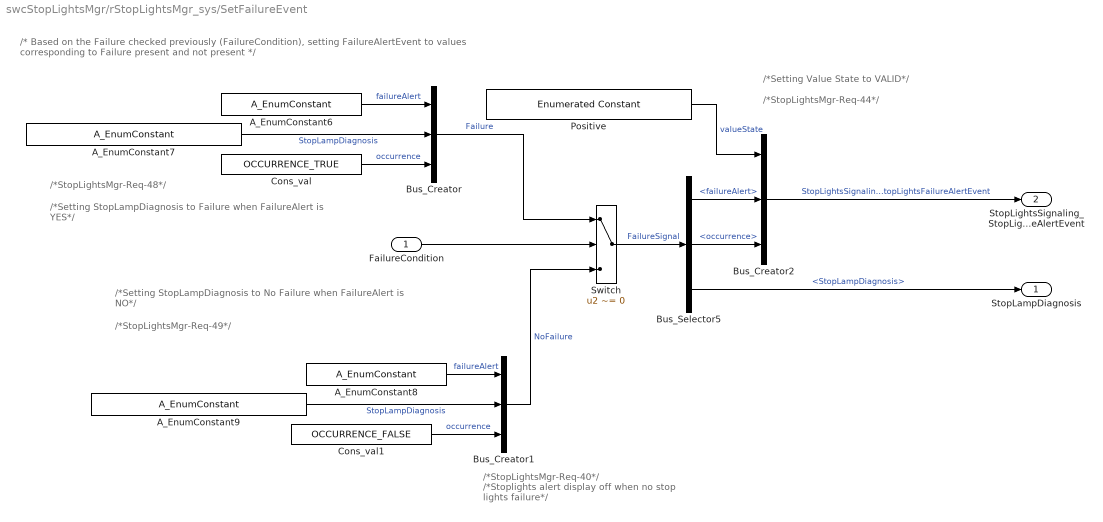
== system swcStopLightsMgr/rStopLightsMgr_sys/SetFailureEvent ==
  note: /*Setting Value State to VALID*/
  note: /*Setting StopLampDiagnosis to Failure
      | when FailureAlert is YES*/
  note: /*Stoplights alert display
      | off when no stop lights failure*/
  note: /*StopLightsMgr-Req-40*/
  note: /*StopLightsMgr-Req-44*/
  note: /*StopLightsMgr-Req-48*/
  note: /*StopLightsMgr-Req-49*/
  note: /*Setting StopLampDiagnosis to No Failure
      | when FailureAlert is NO*/
  note: /* Based on the Failure checked previously (FailureCondition), setting FailureAlertEvent to values corresponding to Failure present and not present */
  FailureCondition : Inport
  A_EnumConstant6 : Ampere_Library/User_Defined_Libraries/Sources/A_EnumConstant  Tag=[LIB]  OutDataTypeStr=Enum: FailureAlert  EnumVal=FAILURE_ALERT_YES
      settings: AttributesFormatString=Enum: FailureAlert
  A_EnumConstant7 : Ampere_Library/User_Defined_Libraries/Sources/A_EnumConstant  Tag=[LIB]  OutDataTypeStr=Enum: CANStopLampDiagnosis  EnumVal=CANSTOPLAMPDIAGNOSIS_FAILURE
      settings: AttributesFormatString=Enum: CANStopLampDiagnosis
  A_EnumConstant8 : Ampere_Library/User_Defined_Libraries/Sources/A_EnumConstant  Tag=[LIB]  OutDataTypeStr=Enum: FailureAlert  EnumVal=FAILURE_ALERT_NO
      settings: AttributesFormatString=Enum: FailureAlert
  A_EnumConstant9 : Ampere_Library/User_Defined_Libraries/Sources/A_EnumConstant  Tag=[LIB]  OutDataTypeStr=Enum: CANStopLampDiagnosis  EnumVal=CANSTOPLAMPDIAGNOSIS_NO_FAILURE
      settings: AttributesFormatString=Enum: CANStopLampDiagnosis
  Bus_Creator : BusCreator  Inputs=failureAlert,StopLampDiagnosis,occurrence
  Bus_Creator1 : BusCreator  Inputs=failureAlert,StopLampDiagnosis,occurrence
  Bus_Creator2 : BusCreator  Inputs=valueState,failureAlert,occurrence  OutDataTypeStr=Bus: StopLightsFailureAlertEvent  NonVirtualBus=on
  Bus_Selector5 : BusSelector  OutputSignals=failureAlert,occurrence,StopLampDiagnosis
  Cons_val : Constant  Value=OCCURRENCE_TRUE
  Cons_val1 : Constant  Value=OCCURRENCE_FALSE
  Positive : simulink/Sources/Enumerated Constant  OutDataTypeStr=Enum: ValueState  Value=ValueState.VALUE_STATE_VALID  SampleTime=inf
      settings: AttributesFormatString=Enum
  Switch : Switch  Criteria=u2 ~= 0  RndMeth=Zero  SaturateOnIntegerOverflow=off
  StopLampDiagnosis : Outport
  StopLightsSignaling_StopLightsFailureAlertEvent : Outport  Port=2
  wires:
  Bus_Creator2/1 -> StopLightsSignaling_StopLightsFailureAlertEvent/1  "StopLightsSignaling_StopLightsFailureAlertEvent"
  FailureCondition/1 -> Switch/2
  A_EnumConstant6/1 -> Bus_Creator/1  "failureAlert"
  Bus_Selector5/2 -> Bus_Creator2/3  "<occurrence>"
  Cons_val1/1 -> Bus_Creator1/3  "occurrence"
  Cons_val/1 -> Bus_Creator/3  "occurrence"
  Bus_Creator/1 -> Switch/1  "Failure"
  Positive/1 -> Bus_Creator2/1  "valueState"
  Switch/1 -> Bus_Selector5/1  "FailureSignal"
  A_EnumConstant9/1 -> Bus_Creator1/2  "StopLampDiagnosis"
  A_EnumConstant7/1 -> Bus_Creator/2  "StopLampDiagnosis"
  Bus_Selector5/1 -> Bus_Creator2/2  "<failureAlert>"
  Bus_Selector5/3 -> StopLampDiagnosis/1  "<StopLampDiagnosis>"
  A_EnumConstant8/1 -> Bus_Creator1/1  "failureAlert"
  Bus_Creator1/1 -> Switch/3  "NoFailure"

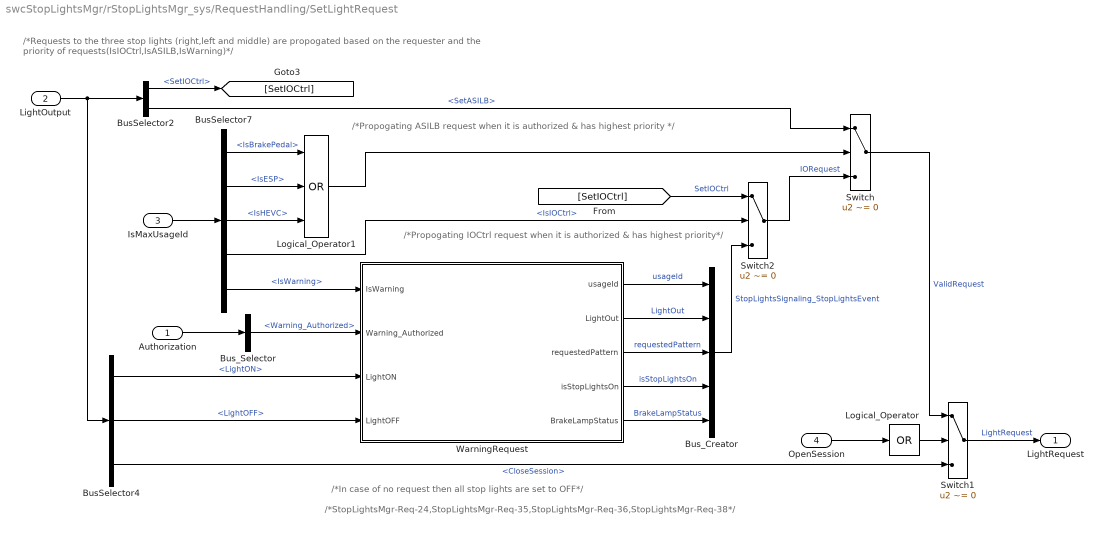
== system swcStopLightsMgr/rStopLightsMgr_sys/RequestHandling/SetLightRequest ==
  note: /*In case of no request then all stop lights are set to OFF*/
  note: /*StopLightsMgr-Req-24,StopLightsMgr-Req-35,StopLightsMgr-Req-36,StopLightsMgr-Req-38*/
  note: /*Propogating IOCtrl request when it is authorized & has highest priority*/
  note: /*Requests to the three stop lights (right,left and middle) are propogated based on the requester and the priority of requests(IsIOCtrl,IsASILB,IsWarning)*/
  note: /*Propogating ASILB request when it is authorized & has highest priority */
  Authorization : Inport
  LightOutput : Inport  Port=2
  IsMaxUsageId : Inport  Port=3
  OpenSession : Inport  Port=4
  BusSelector2 : BusSelector  OutputSignals=SetIOCtrl,SetASILB
  BusSelector4 : BusSelector  OutputSignals=LightBus.LightON,LightBus.LightOFF,LightBus.CloseSession
  BusSelector7 : BusSelector  OutputSignals=IsBrakePedal,IsESP,IsHEVC,IsIOCtrl,IsWarning
  Bus_Creator : BusCreator  Inputs=5  OutDataTypeStr=Bus: lightOutput  NonVirtualBus=on
  Bus_Selector : BusSelector  OutputSignals=Warning_Authorized
  Logical_Operator : Logic  Operator=OR  Inputs=1  OutDataTypeStr=boolean
  Logical_Operator1 : Logic  Operator=OR  Inputs=3  OutDataTypeStr=boolean
  Switch : Switch  Criteria=u2 ~= 0  RndMeth=Zero  SaturateOnIntegerOverflow=off
  Switch1 : Switch  Criteria=u2 ~= 0  RndMeth=Zero  SaturateOnIntegerOverflow=off
  Switch2 : Switch  Criteria=u2 ~= 0  RndMeth=Zero  SaturateOnIntegerOverflow=off
  WarningRequest : Stateflow chart  Description=<binary blob, 133 chars, not shown>  TreatAsAtomicUnit=on
      settings: PortSchema="{\"entries\":[{\"content\":{\"sides\":[{\"content\":{\"connectorIds\":[\"In2\",\"In1\",\"In3\",\"In4\"]},\"type\":\"ConnectorPlacement.EquallySpacedRectSide\",\"uuid\":\"9519dd60-f549-445b-b498-28329e9e4d59\"},{\"content\":{\"connectorIds\":[\"Out1\",\"Out2\",\"Out3\",\"Out4\",\"Out5\"],\"side\":\"RIGHT\"},\"type\":\"ConnectorPlacement.EquallySpacedRectSide\",\"uuid\":\"c2b8f5f7-a152-4150-bb9b-226f7866c343\"},{\"content\":{\"connectorIds\":[],\"side\":\"TOP\"},\"type\":\"ConnectorPlacement.EquallySpacedRectSide\",\"uuid\":\"3024f85f-f443-4f6b-b6a9-525fe81d8a24\"}]},\"type\":\"ConnectorPlacement.EquallySpacedConnector\",\"uuid\":\"41f183e0-a2c2-44a0-9073-9fc493bda50a\"}],\"packageUris\":[\"http://schema.mathworks.com/mf0/Connector/R2020b\"],\"version\":\"1.0\"}"
  LightRequest : Outport
  wires:
  IsMaxUsageId/1 -> BusSelector7/1
  LightOutput/1 -> BusSelector4/1, BusSelector2/1
  Switch2/1 -> Switch/3  "IORequest"
  BusSelector4/2 -> WarningRequest/4(LightOFF)  "<LightOFF>"
  WarningRequest/1(usageId) -> Bus_Creator/1  "usageId"
  WarningRequest/3(requestedPattern) -> Bus_Creator/3  "requestedPattern"
  Bus_Creator/1 -> Switch2/3  "StopLightsSignaling_StopLightsEvent"
  WarningRequest/2(LightOut) -> Bus_Creator/2  "LightOut"
  [SetIOCtrl] -> Switch2/1  "SetIOCtrl"
  WarningRequest/4(isStopLightsOn) -> Bus_Creator/4  "isStopLightsOn"
  WarningRequest/5(BrakeLampStatus) -> Bus_Creator/5  "BrakeLampStatus"
  BusSelector2/1 -> [SetIOCtrl]  "<SetIOCtrl>"
  BusSelector2/2 -> Switch/1  "<SetASILB>"
  BusSelector7/4 -> Switch2/2  "<IsIOCtrl>"
  Authorization/1 -> Bus_Selector/1
  BusSelector4/1 -> WarningRequest/3(LightON)  "<LightON>"
  Bus_Selector/1 -> WarningRequest/1(Warning_Authorized)  "<Warning_Authorized>"
  OpenSession/1 -> Logical_Operator/1
  Logical_Operator/1 -> Switch1/2
  Switch1/1 -> LightRequest/1  "LightRequest"
  Switch/1 -> Switch1/1  "ValidRequest"
  BusSelector4/3 -> Switch1/3  "<CloseSession>"
  BusSelector7/5 -> WarningRequest/2(IsWarning)  "<IsWarning>"
  BusSelector7/3 -> Logical_Operator1/3  "<IsHEVC>"
  BusSelector7/2 -> Logical_Operator1/2  "<IsESP>"
  BusSelector7/1 -> Logical_Operator1/1  "<IsBrakePedal>"
  Logical_Operator1/1 -> Switch/2

== system swcStopLightsMgr/rStopLightsMgr_sys/RequestHandling/SettingLightOutput ==
  note: /*Setting values for LightsON (ASILB & IOControl) and Lights OFF in a bus created locally for reusability in other parts of implementation*/
  Authorization : Inport
  IsMaxUsageId : Inport  Port=2
  BusCreator : BusCreator  Inputs=3
  Bus_Selector : BusSelector  OutputSignals=InputBus
  SetLight : Subsystem
  SetStopLights_ASILB : Subsystem
  SetStopLights_IO : Subsystem
  LightOutput : Outport
  wires:
  BusCreator/1 -> LightOutput/1  "LightOutput"
  SetStopLights_ASILB/1(SetASILB) -> BusCreator/2  "SetASILB"
  SetStopLights_IO/1(SetIOCtrl) -> BusCreator/3  "SetIOCtrl"
  SetLight/1(LightBus) -> SetStopLights_IO/2(LightBus), BusCreator/1, SetStopLights_ASILB/1(LightBus)  "LightBus"
  Authorization/1 -> Bus_Selector/1
  Bus_Selector/1 -> SetStopLights_ASILB/3(InputBus), SetStopLights_IO/1(InputBus)  "<InputBus>"
  IsMaxUsageId/1 -> SetStopLights_ASILB/2(IsMaxUsageId)

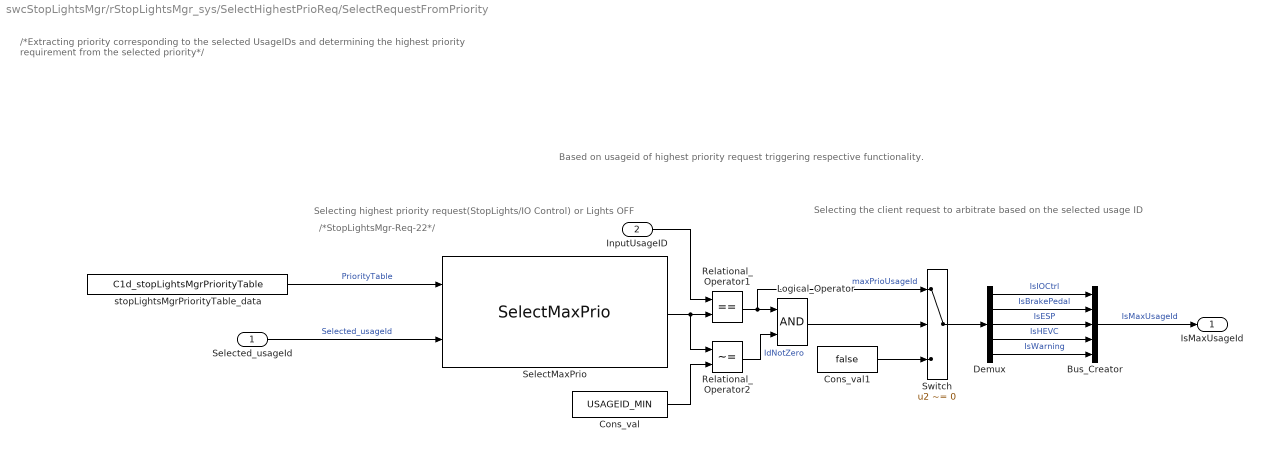
== system swcStopLightsMgr/rStopLightsMgr_sys/SelectHighestPrioReq/SelectRequestFromPriority ==
  note: /*StopLightsMgr-Req-22*/
  note: Selecting the client request to arbitrate based on the selected usage ID
  note: Selecting highest priority request(StopLights/IO Control) or Lights OFF
  note: Based on usageid of highest priority request triggering respective functionality.
  note: /*Extracting priority corresponding to the selected UsageIDs and determining the highest priority requirement from the selected priority*/
  Selected_usageId : Inport
  InputUsageID : Inport  Port=2
  Bus_Creator : BusCreator  Inputs=5
  Cons_val : Constant  Value=USAGEID_MIN
  Cons_val1 : Constant  Value=false
  Demux : Demux  Outputs=5
  Logical_Operator : Logic  OutDataTypeStr=boolean
  Relational_Operator1 : RelationalOperator  Operator===  OutDataTypeStr=boolean  RndMeth=Zero
  Relational_Operator2 : RelationalOperator  Operator=~=  OutDataTypeStr=boolean  RndMeth=Zero
  SelectMaxPrio : KPIT_eBody_Lib_Lighting/SelectMaxPrio  Tag=[LIB]
      settings: LibrarySourceBlock=KPIT_eBody_Lib_Lighting/MaxPrioUsageId
  Switch : Switch  Criteria=u2 ~= 0  RndMeth=Zero  SaturateOnIntegerOverflow=off
  stopLightsMgrPriorityTable_data : Constant  Value=C1d_stopLightsMgrPriorityTable  OutDataTypeStr=Bus: UsageIdPrioEntry
      settings: AttributesFormatString=DT = %<OutDataTypeStr>\n
  IsMaxUsageId : Outport
  wires:
  stopLightsMgrPriorityTable_data/1 -> SelectMaxPrio/1  "PriorityTable"
  Selected_usageId/1 -> SelectMaxPrio/2  "Selected_usageId"
  Demux/1 -> Bus_Creator/1  "IsIOCtrl"
  Demux/2 -> Bus_Creator/2  "IsBrakePedal"
  Bus_Creator/1 -> IsMaxUsageId/1  "IsMaxUsageId"
  Logical_Operator/1 -> Switch/2
  Relational_Operator1/1 -> Switch/1, Logical_Operator/1  "maxPrioUsageId"
  SelectMaxPrio/1 -> Relational_Operator2/1, Relational_Operator1/2
  InputUsageID/1 -> Relational_Operator1/1
  Cons_val/1 -> Relational_Operator2/2
  Switch/1 -> Demux/1
  Cons_val1/1 -> Switch/3
  Relational_Operator2/1 -> Logical_Operator/2  "IdNotZero"
  Demux/3 -> Bus_Creator/3  "IsESP"
  Demux/4 -> Bus_Creator/4  "IsHEVC"
  Demux/5 -> Bus_Creator/5  "IsWarning"

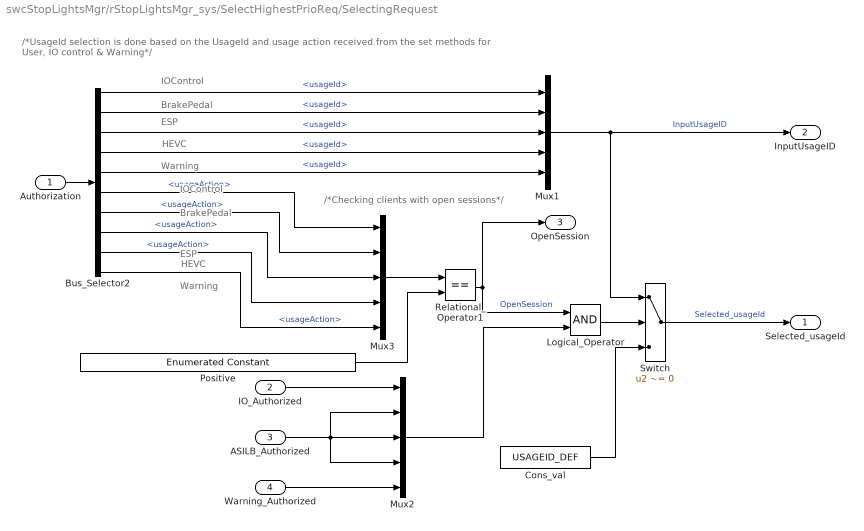
== system swcStopLightsMgr/rStopLightsMgr_sys/SelectHighestPrioReq/SelectingRequest ==
  note: IOControl
  note: /*Checking clients with open sessions*/
  note: /*UsageId selection is done based on the UsageId and usage action received from the set methods for User, IO control & Warning*/
  note: BrakePedal
  note: ESP
  note: HEVC
  note: Warning
  note: HEVC
  note: ESP
  note: Warning
  note: BrakePedal
  note: IOControl
  Authorization : Inport
  IO_Authorized : Inport  Port=2
  ASILB_Authorized : Inport  Port=3
  Warning_Authorized : Inport  Port=4
  Bus_Selector2 : BusSelector  OutputSignals=InputBus.StopLightsDiag_setStopLightsIOControl.usageId,InputBus.BrakePedalStopSignaling_setStopLightsASILB.usageId,InputBus.ElectronicStabilityControlStopSignaling_setStopLightsASILB.usageId,InputBus.RegenerativeBrakingStopSignaling_setStopLightsASILB.usageId,InputBus.OutsideStrongBrakingSignaling_setStopLightsWarningQM.usageId,InputBus.StopLightsDiag_setStopLightsIOControl.usageAction,InputBus.BrakePedalStopSignaling_setStopLightsASILB.usageAction,InputBus.ElectronicStabilityControlStopSignaling_setStopLightsASILB.usageAction,InputBus.RegenerativeBrakingStopSignaling_setStopLightsASILB.usageAction,InputBus.OutsideStrongBrakingSignaling_setStopLightsWarningQM.usageAction
  Cons_val : Constant  Value=USAGEID_DEF
  Logical_Operator : Logic  OutDataTypeStr=boolean
  Mux1 : Mux  Inputs=5
  Mux2 : Mux  Inputs=5
  Mux3 : Mux  Inputs=5
  Positive : simulink/Sources/Enumerated Constant  OutDataTypeStr=Enum: UsageAction  Value=UsageAction.USAGEACTION_OPEN_SESSION  SampleTime=inf
      settings: AttributesFormatString=Enum
  Relational_Operator1 : RelationalOperator  Operator===  OutDataTypeStr=boolean  RndMeth=Zero
  Switch : Switch  Criteria=u2 ~= 0  RndMeth=Zero  SaturateOnIntegerOverflow=off
  Selected_usageId : Outport
  InputUsageID : Outport  Port=2
  OpenSession : Outport  Port=3
  wires:
  Switch/1 -> Selected_usageId/1  "Selected_usageId"
  Mux3/1 -> Relational_Operator1/1
  Positive/1 -> Relational_Operator1/2
  Mux1/1 -> Switch/1, InputUsageID/1  "InputUsageID"
  Cons_val/1 -> Switch/3
  IO_Authorized/1 -> Mux2/1
  ASILB_Authorized/1 -> Mux2/2, Mux2/3, Mux2/4
  Warning_Authorized/1 -> Mux2/5
  Relational_Operator1/1 -> Logical_Operator/1, OpenSession/1  "OpenSession"
  Logical_Operator/1 -> Switch/2
  Mux2/1 -> Logical_Operator/2
  Authorization/1 -> Bus_Selector2/1
  Bus_Selector2/6 -> Mux3/1  "<usageAction>"
  Bus_Selector2/7 -> Mux3/2  "<usageAction>"
  Bus_Selector2/8 -> Mux3/3  "<usageAction>"
  Bus_Selector2/10 -> Mux3/5  "<usageAction>"
  Bus_Selector2/9 -> Mux3/4  "<usageAction>"
  Bus_Selector2/1 -> Mux1/1  "<usageId>"
  Bus_Selector2/2 -> Mux1/2  "<usageId>"
  Bus_Selector2/3 -> Mux1/3  "<usageId>"
  Bus_Selector2/4 -> Mux1/4  "<usageId>"
  Bus_Selector2/5 -> Mux1/5  "<usageId>"

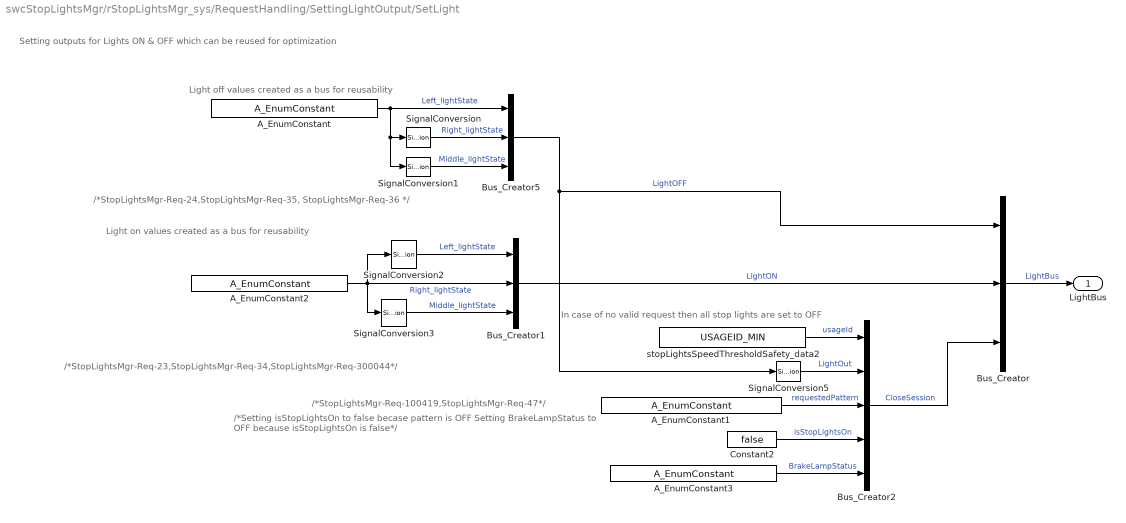
== system swcStopLightsMgr/rStopLightsMgr_sys/RequestHandling/SettingLightOutput/SetLight ==
  note: /*Setting isStopLightsOn to false becase pattern is OFF
      | Setting BrakeLampStatus to OFF because isStopLightsOn is false*/
  note: /*StopLightsMgr-Req-100419,StopLightsMgr-Req-47*/
  note: /*StopLightsMgr-Req-23,StopLightsMgr-Req-34,StopLightsMgr-Req-300044*/
  note: Setting outputs for Lights ON & OFF which can be reused for optimization
  note: Light off values created as a bus for reusability
  note: /*StopLightsMgr-Req-24,StopLightsMgr-Req-35, StopLightsMgr-Req-36 */
  note: Light on values created as a bus for reusability
  note: In case of no valid request then all stop lights are set to OFF
  A_EnumConstant : Ampere_Library/User_Defined_Libraries/Sources/A_EnumConstant  Tag=[LIB]  OutDataTypeStr=Enum: StopLightStateID  EnumVal=STOP_LIGHT_STATE_ID_OFF
      settings: AttributesFormatString=Enum: StopLightStateID
  A_EnumConstant1 : Ampere_Library/User_Defined_Libraries/Sources/A_EnumConstant  Tag=[LIB]  OutDataTypeStr=Enum: StopLightsPatternID  EnumVal=STOP_LIGHTS_PATTERN_ID_OFF
      settings: AttributesFormatString=Enum: StopLightsPatternID
  A_EnumConstant2 : Ampere_Library/User_Defined_Libraries/Sources/A_EnumConstant  Tag=[LIB]  OutDataTypeStr=Enum: StopLightStateID  EnumVal=STOP_LIGHT_STATE_ID_ON
      settings: AttributesFormatString=Enum: StopLightStateID
  A_EnumConstant3 : Ampere_Library/User_Defined_Libraries/Sources/A_EnumConstant  Tag=[LIB]  OutDataTypeStr=Enum: CANBrakeLampStatus  EnumVal=CANBRAKELAMPSTATUS_OFF
      settings: AttributesFormatString=Enum: CANBrakeLampStatus
  Bus_Creator : BusCreator  Inputs=3
  Bus_Creator1 : BusCreator  Inputs='Left_lightState','Right_lightState','Middle_lightState'  OutDataTypeStr=Bus: lightRequest  NonVirtualBus=on
  Bus_Creator2 : BusCreator  Inputs='usageId','LightOut','requestedPattern','isStopLightsOn','BrakeLampStatus'  OutDataTypeStr=Bus: lightOutput  NonVirtualBus=on
  Bus_Creator5 : BusCreator  Inputs=3
  Constant2 : Constant  Value=false
  SignalConversion{,1..3,5} (5 alike) : SignalConversion  OverrideOpt=off
  stopLightsSpeedThresholdSafety_data2 : Constant  Value=USAGEID_MIN
  LightBus : Outport
  wires:
  A_EnumConstant/1 -> Bus_Creator5/1, SignalConversion1/1, SignalConversion/1  "Left_lightState"
  SignalConversion/1 -> Bus_Creator5/2  "Right_lightState"
  SignalConversion1/1 -> Bus_Creator5/3  "Middle_lightState"
  SignalConversion3/1 -> Bus_Creator1/3  "Middle_lightState"
  A_EnumConstant2/1 -> Bus_Creator1/2, SignalConversion2/1, SignalConversion3/1  "Right_lightState"
  SignalConversion2/1 -> Bus_Creator1/1  "Left_lightState"
  Bus_Creator1/1 -> Bus_Creator/2  "LightON"
  Bus_Creator/1 -> LightBus/1  "LightBus"
  Bus_Creator5/1 -> SignalConversion5/1, Bus_Creator/1  "LightOFF"
  stopLightsSpeedThresholdSafety_data2/1 -> Bus_Creator2/1  "usageId"
  SignalConversion5/1 -> Bus_Creator2/2  "LightOut"
  A_EnumConstant1/1 -> Bus_Creator2/3  "requestedPattern"
  A_EnumConstant3/1 -> Bus_Creator2/5  "BrakeLampStatus"
  Bus_Creator2/1 -> Bus_Creator/3  "CloseSession"
  Constant2/1 -> Bus_Creator2/4  "isStopLightsOn"
